simulink model "simulink_ON_OFF_histeresis"  (R2024a)
settings: Solver=VariableStepAuto  StartTime=0.0  StopTime=20  RelTol=1e-3
settings Model: Creator=Monsty  LastModifiedBy=Monsty

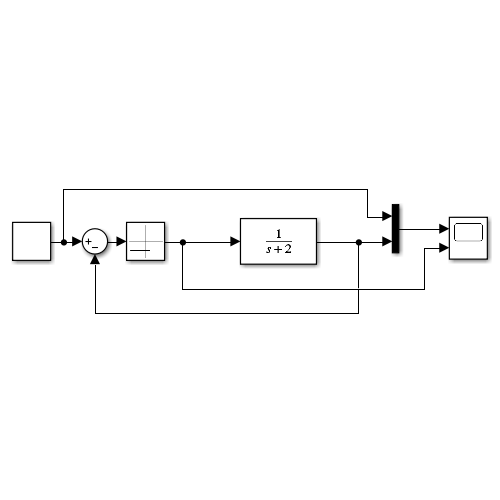
[thumbnail: Simulink's stored preview of the top-level diagram]
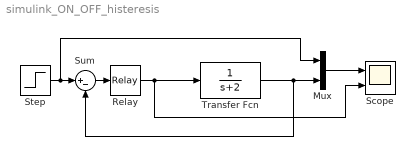
== system simulink_ON_OFF_histeresis ==
  Mux : Mux  Inputs=2
  Relay : Relay  OnSwitchValue=0.1  OffSwitchValue=-0.1  OnOutputValue=10
  Scope : Scope  NumInputPorts=2
  Step : Step  Time=10  Before=1  After=2  SampleTime=0
  Sum : Sum  Inputs=|+-
  Transfer Fcn : TransferFcn  Denominator=[1 2]
  wires:
  Mux/1 -> Scope/1
  Step/1 -> Mux/1, Sum/1
  Transfer Fcn/1 -> Mux/2, Sum/2
  Sum/1 -> Relay/1
  Relay/1 -> Transfer Fcn/1, Scope/2
